simulink model "ToggleOnRisingEdge2"  (R2025a)
settings: Solver=VariableStepAuto  StartTime=0.0  StopTime=10.0  RelTol=1e-3
settings Model: Creator=mahij  LastModifiedBy=mahij

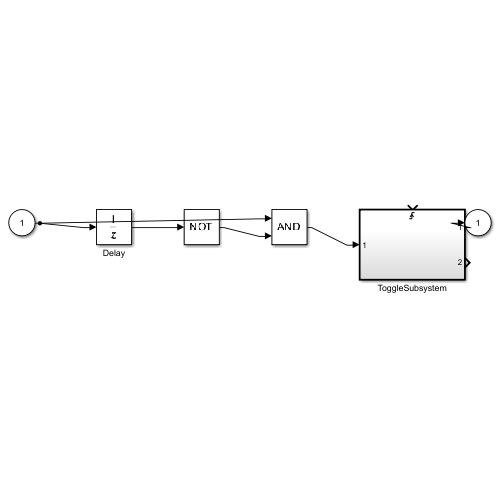
[thumbnail: Simulink's stored preview of the top-level diagram]
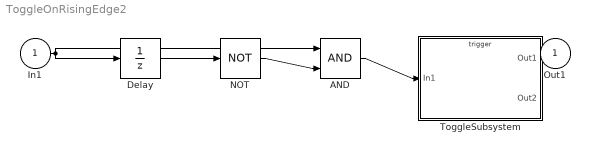
== system ToggleOnRisingEdge2 ==
  In1 : Inport
  AND : Logic  AllPortsSameDT=off  OutDataTypeStr=boolean
  Delay : UnitDelay  SampleTime=-1  HasFrameUpgradeWarning=on
  NOT : Logic  Operator=NOT  AllPortsSameDT=off  OutDataTypeStr=boolean
  ToggleSubsystem : Subsystem  TreatAsAtomicUnit=on
  Out1 : Outport
  wires:
  In1/1 -> Delay/1, AND/1
  Delay/1 -> NOT/1
  NOT/1 -> AND/2
  AND/1 -> ToggleSubsystem/1(In1)
  ToggleSubsystem/1(Out1) -> Out1/1

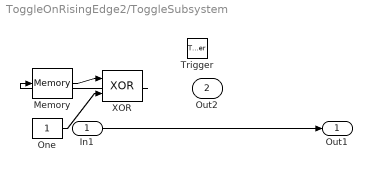
== system ToggleOnRisingEdge2/ToggleSubsystem ==
  In1 : Inport
  Trigger : TriggerPort  VariantControl=(inherit)
  Memory : Memory
  One : Constant
  XOR : Logic  Operator=XOR  AllPortsSameDT=off  OutDataTypeStr=boolean
  Out1 : Outport
  Out2 : Outport  Port=2
  wires:
  In1/1 -> Out1/1
  Memory/1 -> XOR/1
  XOR/1 -> Memory/1
  One/1 -> XOR/2
